simulink model "MATLAB Simulink Model"  (R2020b)
settings: Solver=ode4  StartTime=0.0  StopTime=1  RelTol=1e-3
InitFcn:
  | clear;
  | clc;
  | 
  | %Motor Parameters
  | r1 = 1.405;
  | l1  = 0.005839;
  | r2 = 1.395;
  | l2 = 0.005839;
  | Lm = 0.1722;
  | 
  | %Motor Rated Values
  | Vrat = 400;
  | frat = 50;
  | 
  | x1 = 2*pi*frat*l1;
  | x2 = 2*pi*frat*l2;
  | Xm = 2*pi*frat*Lm;
  | Prat = 4*1000;
  | Nrat = 1430;
  | Ns = 120*frat/4;
  | nrat = Nrat*2*pi/60;
  | ns = Ns*2*pi/60;
  | srat = (Ns-Nrat)/Ns;
  | 
  | E1 = Vrat/sqrt(3); %phase voltage
  | IL = E1/( (r1 + (1i*x1) ) + ( ( (1i*x2) +(r2/srat) )*1i*Xm / ( (1i*Xm) + (1i*x2) + (r2/srat) ) ) );
  | E2 = E1 - (IL*(r1 + (1i*x1) ) );
  | Trat = (3/(ns))*srat*abs(E2)*abs(E2)*r2/((r2*r2) + (srat*srat*x2*x2));
  | %Trat = Prat/nrat;
  | 
  | %System Variables
  | Tsys = (1e-6);
  | Ts = (100e-6);
  | freq = 50;
  | 
  | m=1*freq/50;
  | %m = 1 * (freq/50);
  | Vbus = (400*sqrt(2)*2/sqrt(3)) / (1.15);
  | 
  | Vref = (Vbus*sqrt(3)/2) * m;
  | delay = Ts/Tsys;
  | 
  | % Motor Starting Parameters
  | inc_time = 0.1;
  | 
  | %Motor Loading time
  | load_time = 0.5;
  | 
  | %No. of Hybrid Zones
  | numzones = 3;
  | 
  | %Load ML model Weights
  | 
  | W1R_s1 = readmatrix('Regression Weights\W1_subnet1_tmp_odd_90.xlsx');
  | b1R_s1 = readmatrix('Regression Weights\b1_subnet1_tmp_odd_90.xlsx');
  | W1R_s2 = readmatrix('Regression Weights\W1_subnet2_tmp_odd_90.xlsx');
  | b1R_s2 = readmatrix('Regression Weights\b1_subnet2_tmp_odd_90.xlsx');
  | 
  | W2R = readmatrix('Regression Weights\W2_subnet_tmp_odd_90.xlsx');
  | b2R = readmatrix('Regression Weights\b2_subnet_tmp_odd_90.xlsx');
  | ... (+9 lines)
libraries: powerlib x72, simulink x55, powerlib_meascontrol x15, dspstat3 x11, dspsigops x1
(part 4 of 5)

== system MATLAB Simulink Model/Space Vector PWM based VSI 1/Gating Pulse Generator/Gate Pulse Generator for 2721 Sequence/For Even Sector ==
  "S1, S3, S5" : Inport
  AND : Logic  IconShape=distinctive  AllPortsSameDT=off  OutDataTypeStr=boolean
  AND1 : Logic  IconShape=distinctive  AllPortsSameDT=off  OutDataTypeStr=boolean
  AND2 : Logic  IconShape=distinctive  AllPortsSameDT=off  OutDataTypeStr=boolean
  Carrier1 : simulink/Sources/Repeating Sequence  rep_seq_t=[0 Ts/2 Ts]  rep_seq_y=[Ts-(1e-16) 0 Ts-(1e-16)]
  Carrier2 : simulink/Sources/Repeating Sequence  rep_seq_t=[0 Ts/2 Ts]  rep_seq_y=[0 Ts-(1e-16) 0]
  Constant : Constant
  Constant1 : Constant  Value=2
  Constant2 : Constant  Value=3
  Demux : Demux  Outputs=3
  GreaterThan{,1..3} (4 alike) : RelationalOperator  OutDataTypeStr=boolean  RndMeth=Simplest
  GreaterThan4 : RelationalOperator  Operator===  OutDataTypeStr=boolean  RndMeth=Simplest
  GreaterThan5 : RelationalOperator  Operator===  OutDataTypeStr=boolean  RndMeth=Simplest
  GreaterThan6 : RelationalOperator  Operator===  OutDataTypeStr=boolean  RndMeth=Simplest
  MATLAB Function : MATLAB Function  TreatAsAtomicUnit=on
  XOR : Logic  Operator=XOR  IconShape=distinctive  AllPortsSameDT=off  OutDataTypeStr=boolean
  XOR1 : Logic  Operator=XOR  IconShape=distinctive  AllPortsSameDT=off  OutDataTypeStr=boolean
  XOR2 : Logic  Operator=XOR  IconShape=distinctive  AllPortsSameDT=off  OutDataTypeStr=boolean
  Gate 1 Pulse : Outport
  Gate 3 Pulse : Outport  Port=2
  Gate 5 Pulse : Outport  Port=3
  wires:
  Constant1/1 -> GreaterThan5/1
  AND2/1 -> XOR2/2
  MATLAB Function/3(S5) -> GreaterThan2/1
  XOR1/1 -> Gate 3 Pulse/1
  GreaterThan/1 -> XOR/1
  GreaterThan5/1 -> AND1/2
  MATLAB Function/5(addidx) -> GreaterThan4/2, GreaterThan5/2, GreaterThan6/2
  Constant/1 -> GreaterThan4/1
  Carrier1/1 -> GreaterThan2/2, GreaterThan1/2, GreaterThan/2
  XOR/1 -> Gate 1 Pulse/1
  MATLAB Function/4(addtime) -> GreaterThan3/1
  MATLAB Function/2(S3) -> GreaterThan1/1
  AND1/1 -> XOR1/2
  Constant2/1 -> GreaterThan6/1
  GreaterThan4/1 -> AND/2
  GreaterThan3/1 -> AND2/1, AND1/1, AND/1
  GreaterThan1/1 -> XOR1/1
  GreaterThan6/1 -> AND2/2
  XOR2/1 -> Gate 5 Pulse/1
  Carrier2/1 -> GreaterThan3/2
  Demux/3 -> MATLAB Function/3("S5 ")
  Demux/2 -> MATLAB Function/2("S3 ")
  Demux/1 -> MATLAB Function/1("S1 ")
  MATLAB Function/1(S1) -> GreaterThan/1
  "S1, S3, S5"/1 -> Demux/1
  GreaterThan2/1 -> XOR2/1
  AND/1 -> XOR/2

== system MATLAB Simulink Model/Space Vector PWM based VSI 1/Gating Pulse Generator/Gate Pulse Generator for 2721 Sequence/For Odd Sector ==
  "S1, S3, S1" : Inport
  AND3 : Logic  IconShape=distinctive  AllPortsSameDT=off  OutDataTypeStr=boolean
  AND4 : Logic  IconShape=distinctive  AllPortsSameDT=off  OutDataTypeStr=boolean
  AND5 : Logic  IconShape=distinctive  AllPortsSameDT=off  OutDataTypeStr=boolean
  Carrier3 : simulink/Sources/Repeating Sequence  rep_seq_t=[0 Ts/2 Ts]  rep_seq_y=[0 Ts-(1e-16) 0]
  Constant3 : Constant
  Constant4 : Constant  Value=2
  Constant5 : Constant  Value=3
  Demux1 : Demux  Outputs=3
  GreaterThan{7..10} (4 alike) : RelationalOperator  OutDataTypeStr=boolean  RndMeth=Simplest
  GreaterThan11 : RelationalOperator  Operator===  OutDataTypeStr=boolean  RndMeth=Simplest
  GreaterThan12 : RelationalOperator  Operator===  OutDataTypeStr=boolean  RndMeth=Simplest
  GreaterThan13 : RelationalOperator  Operator===  OutDataTypeStr=boolean  RndMeth=Simplest
  MATLAB Function1 : MATLAB Function  TreatAsAtomicUnit=on
  XOR3 : Logic  Operator=XOR  IconShape=distinctive  AllPortsSameDT=off  OutDataTypeStr=boolean
  XOR4 : Logic  Operator=XOR  IconShape=distinctive  AllPortsSameDT=off  OutDataTypeStr=boolean
  XOR5 : Logic  Operator=XOR  IconShape=distinctive  AllPortsSameDT=off  OutDataTypeStr=boolean
  Gate 1 Pulse : Outport
  Gate 3 Pulse : Outport  Port=2
  Gate 5 Pulse : Outport  Port=3
  wires:
  MATLAB Function1/4(subtime) -> GreaterThan10/1
  Carrier3/1 -> GreaterThan9/2, GreaterThan10/2, GreaterThan8/2, GreaterThan7/2
  "S1, S3, S1"/1 -> Demux1/1
  XOR3/1 -> Gate 1 Pulse/1
  Constant3/1 -> GreaterThan11/1
  XOR5/1 -> Gate 5 Pulse/1
  Demux1/3 -> MATLAB Function1/3("S5 ")
  XOR4/1 -> Gate 3 Pulse/1
  GreaterThan7/1 -> XOR3/1
  Constant5/1 -> GreaterThan13/1
  GreaterThan13/1 -> AND5/2
  GreaterThan8/1 -> XOR4/1
  MATLAB Function1/1(S1) -> GreaterThan7/1
  AND3/1 -> XOR3/2
  GreaterThan11/1 -> AND3/2
  Demux1/1 -> MATLAB Function1/1("S1 ")
  AND4/1 -> XOR4/2
  Demux1/2 -> MATLAB Function1/2("S3 ")
  AND5/1 -> XOR5/2
  MATLAB Function1/2(S3) -> GreaterThan8/1
  MATLAB Function1/5(subidx) -> GreaterThan11/2, GreaterThan12/2, GreaterThan13/2
  GreaterThan10/1 -> AND5/1, AND4/1, AND3/1
  MATLAB Function1/3(S5) -> GreaterThan9/1
  Constant4/1 -> GreaterThan12/1
  GreaterThan9/1 -> XOR5/1
  GreaterThan12/1 -> AND4/2

== system MATLAB Simulink Model/Space Vector PWM based VSI 1/Gating Pulse Generator/Gate Pulse Generator for 7212 Sequence/For Even Sector ==
  "S1, S3, S1" : Inport
  AND3 : Logic  IconShape=distinctive  AllPortsSameDT=off  OutDataTypeStr=boolean
  AND4 : Logic  IconShape=distinctive  AllPortsSameDT=off  OutDataTypeStr=boolean
  AND5 : Logic  IconShape=distinctive  AllPortsSameDT=off  OutDataTypeStr=boolean
  Carrier3 : simulink/Sources/Repeating Sequence  rep_seq_t=[0 Ts/2 Ts]  rep_seq_y=[Ts-(1e-16) 0 Ts-(1e-16)]
  Constant3 : Constant
  Constant4 : Constant  Value=2
  Constant5 : Constant  Value=3
  Demux1 : Demux  Outputs=3
  GreaterThan{7..10} (4 alike) : RelationalOperator  OutDataTypeStr=boolean  RndMeth=Simplest
  GreaterThan11 : RelationalOperator  Operator===  OutDataTypeStr=boolean  RndMeth=Simplest
  GreaterThan12 : RelationalOperator  Operator===  OutDataTypeStr=boolean  RndMeth=Simplest
  GreaterThan13 : RelationalOperator  Operator===  OutDataTypeStr=boolean  RndMeth=Simplest
  MATLAB Function1 : MATLAB Function  TreatAsAtomicUnit=on
  XOR3 : Logic  Operator=XOR  IconShape=distinctive  AllPortsSameDT=off  OutDataTypeStr=boolean
  XOR4 : Logic  Operator=XOR  IconShape=distinctive  AllPortsSameDT=off  OutDataTypeStr=boolean
  XOR5 : Logic  Operator=XOR  IconShape=distinctive  AllPortsSameDT=off  OutDataTypeStr=boolean
  Gate 1 Pulse : Outport
  Gate 3 Pulse : Outport  Port=2
  Gate 5 Pulse : Outport  Port=3
  wires:
  GreaterThan12/1 -> AND4/2
  Carrier3/1 -> GreaterThan9/2, GreaterThan10/2, GreaterThan8/2, GreaterThan7/2
  "S1, S3, S1"/1 -> Demux1/1
  GreaterThan9/1 -> XOR5/1
  Constant4/1 -> GreaterThan12/1
  GreaterThan10/1 -> AND5/1, AND4/1, AND3/1
  MATLAB Function1/1(S1) -> GreaterThan7/1
  MATLAB Function1/3(S5) -> GreaterThan9/1
  MATLAB Function1/5(subidx) -> GreaterThan11/2, GreaterThan12/2, GreaterThan13/2
  Demux1/1 -> MATLAB Function1/1("S1 ")
  MATLAB Function1/2(S3) -> GreaterThan8/1
  Constant3/1 -> GreaterThan11/1
  Constant5/1 -> GreaterThan13/1
  GreaterThan13/1 -> AND5/2
  AND5/1 -> XOR5/2
  MATLAB Function1/4(subtime) -> GreaterThan10/1
  AND3/1 -> XOR3/2
  AND4/1 -> XOR4/2
  XOR4/1 -> Gate 3 Pulse/1
  GreaterThan8/1 -> XOR4/1
  Demux1/2 -> MATLAB Function1/2("S3 ")
  GreaterThan11/1 -> AND3/2
  GreaterThan7/1 -> XOR3/1
  Demux1/3 -> MATLAB Function1/3("S5 ")
  XOR5/1 -> Gate 5 Pulse/1
  XOR3/1 -> Gate 1 Pulse/1

== system MATLAB Simulink Model/Space Vector PWM based VSI 1/Gating Pulse Generator/Gate Pulse Generator for 7212 Sequence/For Odd Sector ==
  "S1, S3, S5" : Inport
  AND : Logic  IconShape=distinctive  AllPortsSameDT=off  OutDataTypeStr=boolean
  AND1 : Logic  IconShape=distinctive  AllPortsSameDT=off  OutDataTypeStr=boolean
  AND2 : Logic  IconShape=distinctive  AllPortsSameDT=off  OutDataTypeStr=boolean
  Carrier1 : simulink/Sources/Repeating Sequence  rep_seq_t=[0 Ts/2 Ts]  rep_seq_y=[0 Ts-(1e-16) 0]
  Carrier2 : simulink/Sources/Repeating Sequence  rep_seq_t=[0 Ts/2 Ts]  rep_seq_y=[Ts-(1e-16) 0 Ts-(1e-16)]
  Constant : Constant
  Constant1 : Constant  Value=2
  Constant2 : Constant  Value=3
  Demux : Demux  Outputs=3
  GreaterThan{,1..3} (4 alike) : RelationalOperator  OutDataTypeStr=boolean  RndMeth=Simplest
  GreaterThan4 : RelationalOperator  Operator===  OutDataTypeStr=boolean  RndMeth=Simplest
  GreaterThan5 : RelationalOperator  Operator===  OutDataTypeStr=boolean  RndMeth=Simplest
  GreaterThan6 : RelationalOperator  Operator===  OutDataTypeStr=boolean  RndMeth=Simplest
  MATLAB Function : MATLAB Function  TreatAsAtomicUnit=on
  XOR : Logic  Operator=XOR  IconShape=distinctive  AllPortsSameDT=off  OutDataTypeStr=boolean
  XOR1 : Logic  Operator=XOR  IconShape=distinctive  AllPortsSameDT=off  OutDataTypeStr=boolean
  XOR2 : Logic  Operator=XOR  IconShape=distinctive  AllPortsSameDT=off  OutDataTypeStr=boolean
  Gate 1 Pulse : Outport
  Gate 3 Pulse : Outport  Port=2
  Gate 5 Pulse : Outport  Port=3
  wires:
  GreaterThan6/1 -> AND2/2
  Demux/2 -> MATLAB Function/2("S3 ")
  Demux/1 -> MATLAB Function/1("S1 ")
  Demux/3 -> MATLAB Function/3("S5 ")
  MATLAB Function/5(addidx) -> GreaterThan4/2, GreaterThan5/2, GreaterThan6/2
  XOR1/1 -> Gate 3 Pulse/1
  Constant1/1 -> GreaterThan5/1
  AND2/1 -> XOR2/2
  AND/1 -> XOR/2
  "S1, S3, S5"/1 -> Demux/1
  Constant2/1 -> GreaterThan6/1
  GreaterThan5/1 -> AND1/2
  GreaterThan2/1 -> XOR2/1
  Carrier2/1 -> GreaterThan3/2
  MATLAB Function/1(S1) -> GreaterThan/1
  GreaterThan4/1 -> AND/2
  XOR2/1 -> Gate 5 Pulse/1
  GreaterThan1/1 -> XOR1/1
  GreaterThan3/1 -> AND2/1, AND1/1, AND/1
  AND1/1 -> XOR1/2
  GreaterThan/1 -> XOR/1
  MATLAB Function/4(addtime) -> GreaterThan3/1
  Constant/1 -> GreaterThan4/1
  MATLAB Function/3(S5) -> GreaterThan2/1
  XOR/1 -> Gate 1 Pulse/1
  MATLAB Function/2(S3) -> GreaterThan1/1
  Carrier1/1 -> GreaterThan2/2, GreaterThan1/2, GreaterThan/2

== matlab function MATLAB Simulink Model/3 Phase Induction Machine/Angle Calculation/MATLAB Function ==
  data: wold input; wnew output; wTs input
function wnew = fcn(wold, wTs)
    wnew = rem(wold + wTs, 2*pi);
end

== matlab function MATLAB Simulink Model/Space Vector PWM based VSI /Gate Pulse Generator/Gate Pulse Values ==
  data: count output; count input; G1 output size=1; S1 input; S3 input; S5 input; G3 output size=1; G5 output size=1; Ts input; Tsys input
function [count, G1, G3, G5] = fcn(count, S1, S3, S5, Ts, Tsys)
    count = double(rem(int32(1+count), int32(Ts/Tsys)));
    G1 = S1(1+count);
    G3 = S3(1+count);
    G5 = S5(1+count);
    
%     G1=S1;
%     G3= S3;
%     G5 = S5;
end

== matlab function MATLAB Simulink Model/Space Vector PWM based VSI /Gating Pulse Generator/Gate Pulse Generator for 0127 Sequence 1/For Odd Sector/MATLAB Function1 ==
  data: S1 input; S1 output; S3 input; S5 input; S3 output; S5 output; subtime output; subidx output
function [S1, S3, S5, subtime,subidx] = fcn(S1, S3, S5)
    S = [S1 S3 S5];
    [~, idx] = mink([S1 S3 S5], 3);
    
    subtime = ( ( S(idx(2)) - S(idx(1)) )/2);
    S(idx(1)) = S(idx(1)) + subtime;
    subidx = idx(1);
    
    S1 = S(1);
    S3 = S(2);
    S5 = S(3);
end

== matlab function MATLAB Simulink Model/Space Vector PWM based VSI /Gating Pulse Generator/Gate Pulse Generator for 7212 Sequence/For Even Sector/MATLAB Function1 ==
  data: S1 input; S1 output; S3 input; S5 input; S3 output; S5 output; subtime output; subidx output
function [S1, S3, S5, subtime,subidx] = fcn(S1, S3, S5)
    S = [S1 S3 S5];
    [~, idx] = mink([S1 S3 S5], 3);
    
    S(idx(2)) = (S(idx(2)) + S(idx(3)))/2;
    
    subidx = idx(2);
    subtime = S(idx(3)) - S(idx(2));
    
    S1 = S(1);
    S3 = S(2);
    S5 = S(3);
end

== matlab function MATLAB Simulink Model/Space Vector PWM based VSI /Gating Pulse Generator/Gate Pulse Generator for 0121 Sequence/For Even Sector/MATLAB Function ==
  data: S1 input; S1 output; S3 input; S5 input; S3 output; S5 output; addtime output; addidx output
function [S1, S3, S5, addtime,addidx] = fcn(S1, S3, S5)
    S = [S1 S3 S5];
    [~, idx] = mink([S1 S3 S5], 3);
    
    addtime = (S(idx(2)) - S(idx(1)))/2;
    addidx = idx(2);
    S(idx(2)) = S(idx(2)) - addtime;
    
    S1 = S(1);
    S3 = S(2);
    S5 = S(3);
end

== matlab function MATLAB Simulink Model/Space Vector PWM based VSI /Switching Times and Sector/Switch Times and Sequence Calculation ==
  data: Vref input; angle input; Ts input; Vbus input; sector output
function sector  = fcn(Vref, angle, Ts, Vbus)
    
    numzones = 3;
    %     Using ML Models 
    m = (2/sqrt(3))*(Vref/Vbus);
    theta = rem(angle, (pi/3));
    flag = 0;
    if numzones == 1
        flag = 1;
    end
    
    %Switching times calculation of different vectors
    if m <= 1                % Linear modulation (Overmodulation mode 0)
        n2 = Vref*cos( theta );
        n1 = Vref*cos( (pi/3) - theta );

        T1 = (2*Ts/(3*Vbus)) * ((-n1) + (2*n2));
        T2 = (2*Ts/(3*Vbus)) * ((2*n1) - n2);
        T0 = Ts-(T1+T2);
        flag = 1;
        
    elseif m<=1.05      % Overmodulation mode I
        alpha_t = (pi/6) - acos(1/m);
        alpha_t = alpha_t/2;
        if theta > alpha_t && theta < (pi/3) - alpha_t
            T1 = (sin( (pi/3) - theta ) / ( sin( (pi/3) - theta ) + sin( theta ) ) ) * Ts;
            T2 = Ts-T1;
            T0=0;
        else
            n2 = Vref*cos( theta );
            n1 = Vref*cos( (pi/3) - theta );
            T1 = (2*Ts/(3*Vbus)) * ((-n1) + (2*n2));
            T2 = (2*Ts/(3*Vbus)) * ((2*n1) - n2);
            T0 = Ts-(T1+T2);
            flag = 1;
        end
        
    elseif m <= 1.10    % Overmodulation mode II
        alpha_h = (pi/6) - acos(1/m);
        if theta <= alpha_h
            T1 = Ts;
            T2=0;
            T0=0;
            
        elseif theta > alpha_h && theta < (pi/3) - alpha_h
            T1 = (sin( (pi/3) - theta ) / ( sin( (pi/3) - theta ) + sin( theta ) ) ) * Ts;
            T2 = Ts-T1;
            T0=0;
            
        else
            T1 = 0;
            T2 = Ts;
            T0 = 0;
        end
        
    else        % Six Step Mode
        if theta <= (pi/6)
            T1 = Ts;
            T2 = 0;
            T0 = 0;
        else
            T1 = 0;
            T2 = Ts;
            T0 = 0;
        end
        
    end
    
    if flag == 1
        % Switching Sequence Determination
        Q1 = (cos(theta) - (Vref/Vbus)) * T1;
        Q2 = (cos( (pi/3) - theta) - (Vref/Vbus)) * T2;
        Q0 = - (Vref/Vbus)*T0;
        D = sin(theta) * T1;

        %Error Functions (Squared) for Different Switching Sequences
        F_0127 = ( (1/3) * ( (0.5*Q0).^2 ) * T0 / (2*Ts) ) + ( (1/3) * ( ( (0.5*Q0).^2 ) + ( 0.5*Q0* ( (0.5*Q0) + Q1 ) ) + ( ( 1* ( (0.5*Q0) + Q1 ) ).^2) ) * (T1/Ts) ) + ( (1/3) * ( ( ( (0.5*Q0) + Q1).^2) - ( ( (0.5*Q0) + Q1) * (0.5*Q0) ) + ( (0.5*Q0).^2 ) ) * (T2/Ts) ) + ( (1/3) * ( (0.5*Q0).^2 ) * ( T0 / (2*Ts) ) ) + ( (1/3) * (D.^2) * ( (T1+T2) / Ts ) );

        F_012 = ( (4/27) * (Q0.^2) * (T0/Ts) ) + ( (4/27) * ( (Q0.^2) + ( Q0*(Q0+Q1) ) + ( (Q0+Q1).^2 ) ) * (T1/Ts) ) + ( (4/27) * ( (Q0+Q1).^2 ) * (T2/Ts) ) + ( (4/27) * (D.^2) * ( (T1+T2) / Ts) );

        F_721 = ( (4/27) * (Q0.^2) * (T0/Ts) ) + ( (4/27) * ( (Q0.^2) + ( Q0*(Q0+Q2) ) + ( (Q0+Q2).^2 ) ) * (T2/Ts) ) + ( (4/27) * ( (Q0+Q2).^2 ) * (T1/Ts) ) + ( (4/27) * (D.^2) * ( (T1+T2) / Ts) );

        F_0121 = ( (1/3) * (Q0.^2) * (T0/Ts) ) + ( (1/3) * ( (Q0.^2) + ( Q0*( Q0 + (0.5*Q1) ) ) + ( ( Q0 + (0.5*Q1) ).^2 ) ) * ( T1 / (2*Ts) ) ) + ( (1/3) * ( ( ( Q0 + (0.5*Q1) ).^2 ) - ( ( Q0 + (0.5*Q1) ) * (0.5*Q1) ) + ( (0.5*Q1).^2 ) ) * (T2/Ts) ) + ( (1/3) * ( (0.5*Q1).^2 ) * (T1 / (2*Ts) ) ) + ( (1/3) * ( (0.5*D).^2 ) * ( (T1+T2) / Ts ) );

        F_7212 = ( (1/3) * (Q0.^2) * (T0/Ts) ) + ( (1/3) * ( (Q0.^2) + ( Q0*( Q0 + (0.5*Q2) ) ) + ( ( Q0 + (0.5*Q2) ).^2 ) ) * ( T2 / (2*Ts) ) ) + ( (1/3) * ( ( ( Q0 + (0.5*Q2) ).^2 ) - ( ( Q0 + (0.5*Q2) ) * (0.5*Q2) ) + ( (0.5*Q2).^2 ) ) * (T1/Ts) ) + ( (1/3) * ( (0.5*Q2).^2 ) * (T2 / (2*Ts) ) ) + ( (1/3) * ( (0.5*D).^2 ) * ( (T1+T2) / Ts ) );

        F_1012 = ( (1/3) * ( ( 0.5*Q1).^2 ) * (T1 / (2*Ts) ) ) + ( (1/3) * ( ( (0.5*Q1).^2 ) + ( 0.5*Q1*( (0.5*Q1) + Q0 ) ) + ( ( (0.5*Q1) + Q0 ).^2 ) ) * (T0/Ts) ) + ( (1/3) * ( ( ( (0.5*Q1) + Q0 ).^2 ) - ( ( (0.5*Q1) + Q0 )*Q2 ) + (Q2.^2) ) * ( T1 / (2*Ts) ) ) + ( (1/3) * (Q2.^2) * (T2/Ts) ) + ( (1/3) * ( (0.5*D).^2 ) * ( T1 / (2*Ts) ) ) + ( ( (0.5*D).^2 ) * (T0/Ts) ) + ( (1/3) * ( ( (0.5*D).^2 ) + ( (0.5*D) * D ) + (D.^2) ) * ( T1 / (2*Ts) ) ) + ( (1/3) * (D.^2) * (T2/Ts) );

        F_2721 = ( (1/3) * ( ( 0.5*Q2).^2 ) * (T2 / (2*Ts) ) ) + ( (1/3) * ( ( (0.5*Q2).^2 ) + ( 0.5*Q2*( (0.5*Q2) + Q0 ) ) + ( ( (0.5*Q2) + Q0 ).^2 ) ) * (T0/Ts) ) + ( (1/3) * ( ( ( (0.5*Q2) + Q0 ).^2 ) - ( ( (0.5*Q2) + Q0 )*Q1 ) + (Q1.^2) ) * ( T2 / (2*Ts) ) ) + ( (1/3) * (Q1.^2) * (T1/Ts) ) + ( (1/3) * ( (0.5*D).^2 ) * ( T2 / (2*Ts) ) ) + ( ( (0.5*D).^2 ) * (T0/Ts) ) + ( (1/3) * ( ( (0.5*D).^2 ) + ( (0.5*D) * D ) + (D.^2) ) * ( T2 / (2*Ts) ) ) + ( (1/3) * (D.^2) * (T1/Ts) );
        
        if numzones == 1
            F = [F_0127];
            
        elseif numzones == 3
            %For Three Zone Hybrid PWM
            F = [F_0127, F_0121, F_7212];
            
        elseif numzones == 5
            %For Five Zone Hybrid PWM
            F = [F_0127, F_0121, F_7212, F_1012, F_2721];
        
        elseif numzones == 7
            %For Seven Zone Hybrid PWM
            F = [F_0127, F_0121, F_7212, F_1012, F_2721, F_012, F_721];
            
        else
            F = F_0127;
        end
        
        [~, idx] = min(F);

        if idx == 1
            switchseq = "0127";
        elseif idx == 2
            switchseq = "0121";
        elseif idx == 3
            switchseq = "7212";
        elseif idx == 4
            switchseq = "1012";
        elseif idx == 5
            switchseq = "2721";
        elseif idx == 6
            switchseq = "012";
        elseif idx == 7
            switchseq = "721";
        else
            switchseq = "0127";
        end
        
    else
        if theta < (pi/6)
            switchseq = "0121";
        else
            switchseq = "7212";
        end
    end
    
    % Switching Times calculation of switches
    Vsamp = Vref*exp(1i*angle);
    
    V1 = Vbus*exp(1i*0);
    V2 = Vbus*exp(1i*(pi/3));
    V3 = Vbus*exp(1i*(2*pi/3));
    V4 = Vbus*exp(1i*(3*pi/3));
    V5 = Vbus*exp(1i*(4*pi/3));
    V6 = Vbus*exp(1i*(5*pi/3));

    V = [V1; V2; V3; V4; V5; V6];
    V = V - Vsamp;
    [~, minVidx] = mink(V, 2);

%         minVidx = minVidx(:, 1);

    if max(minVidx) == 6 && min(minVidx) == 1
        minVidx = 6;
    else
        minVidx = min(minVidx);
    end
    
    sector = minVidx;
    
    if switchseq == "0127"
        swseq = 1;
    elseif switchseq == "0121"
        swseq = 2;
    elseif switchseq == "7212"
        swseq = 3;
    elseif switchseq == "1012"
        swseq = 4;
    elseif switchseq == "2721"
        swseq = 5;
    elseif switchseq == "012"
        swseq = 6;
    elseif switchseq == "721"
        swseq = 7;
    else
        swseq = 1;
    end
%     
%     %Using NN to predict switch times
%     
%     %Loading Necessary weight matrices
%     W1 = evalin('base', 'W1R');
%     b1 = evalin('base', 'b1R');
%     W2 = evalin('base', 'W2R');
%     b2 = evalin('base', 'W2R');
%     
%     %Predicting Switch Times
%     X = [m angle];
% %     y1 = zeros(1, size(b1, 1));
% %     y2 = zeros(1, size(b2, 2));
%     
%     y = X*(W1');
%     y = y + b1';      %Passing through 1st Layer (Hidden)
%     y = tanh(y);                  %Applying Activation Function (tanh)
%     
%     y = y*W2';
%     y = y+b2';        %Passing through 2nd Layer (Output)
%     y = 1./(1+exp(-y));      %Applying Activation Function (sigmoid)
%     
%     %Allocating Switch Times
%     S1 = y(1)*Ts;
%     S3 = y(2)*Ts;
%     S5 = y(3)*Ts;
    
end

== matlab function MATLAB Simulink Model/Space Vector PWM based VSI /Gating Pulse Generator/Gate Pulse Generator for 1012 Sequence/For Even Sector/MATLAB Function1 ==
  data: S1 input; S1 output; S3 input; S5 input; S3 output; S5 output; subtime output; subidx output
function [S1, S3, S5, subtime,subidx] = fcn(S1, S3, S5)
    S = [S1 S3 S5];
    [~, idx] = mink([S1 S3 S5], 3);
    
    subtime = ( ( S(idx(2)) - S(idx(1)) )/2);
    S(idx(1)) = S(idx(1)) + subtime;
    subidx = idx(1);
    
    S1 = S(1);
    S3 = S(2);
    S5 = S(3);
end

== matlab function MATLAB Simulink Model/Space Vector PWM based VSI /Gating Pulse Generator/Gate Pulse Generator for 0127 Sequence 1/For Even Sector/MATLAB Function ==
  data: S1 input; S1 output; S3 input; S5 input; S3 output; S5 output; addtime output; addidx output
function [S1, S3, S5, addtime,addidx] = fcn(S1, S3, S5)
    S = [S1 S3 S5];
    [~, idx] = mink([S1 S3 S5], 3);
    
    addtime = (S(idx(3)) - S(idx(2)))/2;
    addidx = idx(3);
    S(idx(3)) = S(idx(3)) - addtime;
    
    S1 = S(1);
    S3 = S(2);
    S5 = S(3);
end

== matlab function MATLAB Simulink Model/Space Vector PWM based VSI /Gating Pulse Generator/Gate Pulse Generator for 0121 Sequence/For Odd Sector/MATLAB Function ==
  data: S1 input; S1 output; S3 input; S5 input; S3 output; S5 output; subtime output; subidx output
function [S1, S3, S5, subtime,subidx] = fcn(S1, S3, S5)
    S = [S1 S3 S5];
    [~, idx] = mink([S1 S3 S5], 3);
    
    S(idx(2)) = (S(idx(2)) + S(idx(3)))/2;
    
    subidx = idx(2);
    subtime = S(idx(3)) - S(idx(2));
    
    S1 = S(1);
    S3 = S(2);
    S5 = S(3);
end

== matlab function MATLAB Simulink Model/Space Vector PWM based VSI /Gating Pulse Generator/Gate Pulse Generator for 1012 Sequence/For Odd Sector/MATLAB Function ==
  data: S1 input; S1 output; S3 input; S5 input; S3 output; S5 output; addtime output; addidx output
function [S1, S3, S5, addtime,addidx] = fcn(S1, S3, S5)
    S = [S1 S3 S5];
    [~, idx] = mink([S1 S3 S5], 3);
    
    addtime = (S(idx(3)) - S(idx(2)))/2;
    addidx = idx(3);
    S(idx(3)) = S(idx(3)) - addtime;
    
    S1 = S(1);
    S3 = S(2);
    S5 = S(3);
end

== matlab function MATLAB Simulink Model/Space Vector PWM based VSI /Gating Pulse Generator/Gate Pulse Generator for 2721 Sequence/For Even Sector/MATLAB Function ==
  data: S1 input; S1 output; S3 input; S5 input; S3 output; S5 output; addtime output; addidx output
function [S1, S3, S5, addtime,addidx] = fcn(S1, S3, S5)
    S = [S1 S3 S5];
    [~, idx] = mink([S1 S3 S5], 3);
    
    addtime = (S(idx(3)) - S(idx(2)))/2;
    addidx = idx(3);
    S(idx(3)) = S(idx(3)) - addtime;
    
    S1 = S(1);
    S3 = S(2);
    S5 = S(3);
end

== matlab function MATLAB Simulink Model/15 Hz System/Space Vector PWM based VSI 1/Switching Times and Sector/Switching times of all switches ==
  data: Vref input; S1 output; theta input; Ts input; sector input; S3 output; S5 output; Vbus input
function [S1, S3, S5] = fcn(Vref, theta, Ts, sector, Vbus)
    n2 = Vref*cos(theta);
    n1 = Vref*cos((pi/3)-theta);
    
%     T1 = sqrt(3)*Ts*Vref*(sin(sector*pi/3)*cos(angle - ((sector-1)*pi/3)) - cos(sector*pi/3)*sin(angle - ((sector-1)*pi/3)))/u(3);
%     T2 = sqrt(3)*Ts*Vref*(-cos(angle - ((sector-1)*pi/3))*sin((sector-1)*pi/3) + sin(angle - ((sector-1)*pi/3))*cos((sector-1)*pi/3))/u(3);
    
    T1 = (2*Ts/(3*Vbus)) * ((-n1) + (2*n2));
    T2 = (2*Ts/(3*Vbus)) * ((2*n1) - n2);
    T0 = Ts-(T1+T2);
  
    if sector == 1
        S1 = T1+T2+(T0/2);
%         S4 = T0/2;
        S3 = T2+(T0/2);
%         S6 = T1+(T0/2);
        S5 = T0/2;
%         S2 = T1+T2+(T0/2);
    elseif sector == 2
        S1 = T1+(T0/2);
%         S4 = T2+(T0/2);
        S3 = T1+T2+(T0/2);
%         S6 = (T0/2);
        S5 = T0/2;
%         S2 = T1+T2+(T0/2);
    elseif sector == 3
        S1 = (T0/2);
%         S4 = T1+T2+(T0/2);
        S3 = T1+T2+(T0/2);
%         S6 = (T0/2);
        S5 = T2+(T0/2);
%         S2 = T1+(T0/2);
    elseif sector == 4
        S1 = (T0/2);
%         S4 = T1+T2+(T0/2);
        S3 = T1+(T0/2);
%         S6 = T2+(T0/2);
        S5 = T1+T2+(T0/2);
%         S2 = (T0/2);
    elseif sector == 5
        S1 = T2+(T0/2);
%         S4 = T1+(T0/2);
        S3 = (T0/2);
%         S6 = T1+T2+(T0/2);
        S5 = T1+T2+(T0/2);
%         S2 = (T0/2);
    elseif sector == 6
        S1 = T1+T2+(T0/2);
%         S4 = T0/2;
        S3 = (T0/2);
%         S6 = T1+T2+(T0/2);
        S5 = T1+(T0/2);
%         S2 = T2+(T0/2);
    else
        S1 = (T1+T2+T0)/2;
        S3 = (T1+T2+T0)/2;
        S5 = (T1+T2+T0)/2;
    end
end

== matlab function MATLAB Simulink Model/Space Vector PWM based VSI /Switching Times and Sector/MATLAB Function1 ==
  data: u input; S1 output; S3 output; S5 output
function [S1, S3, S5] = fcn(u)
    S1 = u(1);
    S3 = u(2);
    S5 = u(3);
end

== matlab function MATLAB Simulink Model/Space Vector PWM based VSI /Gating Pulse Generator/Gate Pulse Generator for 7212 Sequence/For Odd Sector/MATLAB Function ==
  data: S1 input; S1 output; S3 input; S5 input; S3 output; S5 output; addtime output; addidx output
function [S1, S3, S5, addtime,addidx] = fcn(S1, S3, S5)
    S = [S1 S3 S5];
    [~, idx] = mink([S1 S3 S5], 3);
    
    addtime = (S(idx(2)) - S(idx(1)))/2;
    addidx = idx(2);
    S(idx(2)) = S(idx(2)) - addtime;
    
    S1 = S(1);
    S3 = S(2);
    S5 = S(3);
end

== matlab function MATLAB Simulink Model/Space Vector PWM based VSI /Gating Pulse Generator/Gate Pulse Generator for 2721 Sequence/For Odd Sector/MATLAB Function1 ==
  data: S1 input; S1 output; S3 input; S5 input; S3 output; S5 output; subtime output; subidx output
function [S1, S3, S5, subtime,subidx] = fcn(S1, S3, S5)
    S = [S1 S3 S5];
    [~, idx] = mink([S1 S3 S5], 3);
    
    subtime = ( ( S(idx(2)) - S(idx(1)) )/2);
    S(idx(1)) = S(idx(1)) + subtime;
    subidx = idx(1);
    
    S1 = S(1);
    S3 = S(2);
    S5 = S(3);
end

== matlab function MATLAB Simulink Model/Space Vector PWM based VSI /Switching Times and Sector/Feature Expand ==
  data: X input; new_X output size=[1 18]
function new_X = fcn(X)
    X = X';
    new_X = zeros(1,18);
    new_X(1, 1) = X(1, 1);
    new_X(1, 2) = X(1, 2);
    
    %Include sinusoidal terms (1st order)
    new_X(1, 3) = sin(X(1, 1));
    new_X(1, 4) = sin(X(1, 2));
    new_X(1, 5) = cos(X(1, 1));
    new_X(1, 6) = cos(X(1, 2));
%     new_X(1, 7) = sin(X(1, 1).*X(1, 2));
%     new_X(1, 8) = cos(X(1, 1).*X(1, 2));
    
%Include 2nd harmonic sinusoidal terms
    new_X(1, 7) = sin(2*X(1, 1));
    new_X(1, 8) = sin(2*X(1, 2));
    new_X(1, 9) = cos(2*X(1, 1));
    new_X(1, 10) = cos(2*X(1, 2));
    
        %Include 3rd harmonic sinusoidal terms
    new_X(1, 11) = sin(3*X(1, 1));
    new_X(1, 12) = sin(3*X(1, 2));
    new_X(1, 13) = cos(3*X(1, 1));
    new_X(1, 14) = cos(3*X(1, 2));
    
    %Include 4th harmonic sinusoidal terms
    new_X(1, 15) = sin(4*X(1, 1));
    new_X(1, 16) = sin(4*X(1, 2));
    new_X(1, 17) = cos(4*X(1, 1));
    new_X(1, 18) = cos(4*X(1, 2));

%     %Include 2nd order terms
%     new_X(:, 3) = X(:, 1).*X(:, 1);
%     new_X(:, 4) = X(:, 1).*X(:, 2);
%     new_X(:, 5) = X(:, 2).*X(:, 2);
    
%     %Include 3rd order terms
%     new_X(:, 6) = X(:, 1).*X(:, 1).*X(:, 1);
%     new_X(:, 7) = X(:, 1).*X(:, 1).*X(:, 2);
%     new_X(:, 8) = X(:, 1).*X(:, 2).*X(:, 2);
%     new_X(:, 9) = X(:, 2).*X(:, 2).*X(:, 2);
%     
%     %Incluce 4th order terms
%     new_X(:, 10) = X(:, 1).*X(:, 1).*X(:, 1).*X(:, 1);
%     new_X(:, 11) = X(:, 1).*X(:, 1).*X(:, 1).*X(:, 2);
%     new_X(:, 12) = X(:, 1).*X(:, 1).*X(:, 2).*X(:, 2);
%     new_X(:, 13) = X(:, 1).*X(:, 2).*X(:, 2).*X(:, 2);
%     new_X(:, 14) = X(:, 2).*X(:, 2).*X(:, 2).*X(:, 2);
%     
%     %Incluce 5th order terms
%     new_X(:, 15) = X(:, 1).*X(:, 1).*X(:, 1).*X(:, 1).*X(:, 1);
%     new_X(:, 16) = X(:, 1).*X(:, 1).*X(:, 1).*X(:, 1).*X(:, 2);
%     new_X(:, 17) = X(:, 1).*X(:, 1).*X(:, 1).*X(:, 2).*X(:, 2);
%     new_X(:, 18) = X(:, 1).*X(:, 1).*X(:, 2).*X(:, 2).*X(:, 2);
%     new_X(:, 19) = X(:, 1).*X(:, 2).*X(:, 2).*X(:, 2).*X(:, 2);
%     new_X(:, 20) = X(:, 2).*X(:, 2).*X(:, 2).*X(:, 2).*X(:, 2);
%     
%     %Incluce 6th order terms
%     new_X(:, 21) = X(:, 1).*X(:, 1).*X(:, 1).*X(:, 1).*X(:, 1).*X(:, 1);
%     new_X(:, 22) = X(:, 1).*X(:, 1).*X(:, 1).*X(:, 1).*X(:, 1).*X(:, 2);
%     new_X(:, 23) = X(:, 1).*X(:, 1).*X(:, 1).*X(:, 1).*X(:, 2).*X(:, 2);
%     new_X(:, 24) = X(:, 1).*X(:, 1).*X(:, 1).*X(:, 2).*X(:, 2).*X(:, 2);
%     new_X(:, 25) = X(:, 1).*X(:, 1).*X(:, 2).*X(:, 2).*X(:, 2).*X(:, 2);
%     new_X(:, 26) = X(:, 1).*X(:, 2).*X(:, 2).*X(:, 2).*X(:, 2).*X(:, 2);
%     new_X(:, 27) = X(:, 2).*X(:, 2).*X(:, 2).*X(:, 2).*X(:, 2).*X(:, 2);
end

== matlab function MATLAB Simulink Model/Space Vector PWM based VSI /Switching Times and Sector/Angle Calculation1/MATLAB Function ==
  data: wold input; wnew output; wTs input
function wnew = fcn(wold, wTs)
    wnew = rem(wold + wTs, 2*pi);
end

== matlab function MATLAB Simulink Model/Space Vector PWM based VSI /Switching Times and Sector/MATLAB Function2 ==
  data: Vref input; V_alpha output; angle input; V_beta output
function [V_alpha, V_beta] = fcn(Vref, angle)
    V_alpha = Vref*cos(angle);
    V_beta = Vref*sin(angle);
end

== matlab function MATLAB Simulink Model/Space Vector PWM based VSI /Switching Times and Sector/MATLAB Function3 ==
  data: u input; u output
function u = fcn(u)
    u(u<0) = 0;
end

== matlab function MATLAB Simulink Model/Space Vector PWM based VSI /3 Phase VSI/MATLAB Function ==
  data: iter input; iter output; arr input size=[1 3]; Va input; Vb input; Vc input; Ts input; Tsys input; arr output
function [iter, arr] = fcn(iter, arr, Va, Vb, Vc, Ts, Tsys)
    if iter == Ts/Tsys
        iter=0;
        arr = zeros(1,3);
    end
    arr(1, 1) = arr(1, 1) + (Va*Tsys/Ts);
    arr(1, 2) = arr(1, 2) + (Vb*Tsys/Ts);
    arr(1, 3) = arr(1, 3) + (Vc*Tsys/Ts);
    iter = iter+1;
end

== matlab function MATLAB Simulink Model/Space Vector PWM based VSI 1/3 Phase VSI/MATLAB Function ==
  data: iter input; iter output; arr input size=[1 3]; Va input; Vb input; Vc input; Ts input; Tsys input; arr output
function [iter, arr] = fcn(iter, arr, Va, Vb, Vc, Ts, Tsys)
    if iter == Ts/Tsys
        iter=0;
        arr = zeros(1,3);
    end
    arr(1, 1) = arr(1, 1) + (Va*Tsys/Ts);
    arr(1, 2) = arr(1, 2) + (Vb*Tsys/Ts);
    arr(1, 3) = arr(1, 3) + (Vc*Tsys/Ts);
    iter = iter+1;
end

== matlab function MATLAB Simulink Model/Space Vector PWM based VSI /Switching Times and Sector/MATLAB Function4 ==
  data: u input; y output
function y = fcn(u)
    [~, y] = max(u);
end

== matlab function MATLAB Simulink Model/Space Vector PWM based VSI 1/Gate Pulse Generator/Gate Pulse Values ==
  data: count output; count input; G1 output size=1; S1 input; S3 input; S5 input; G3 output size=1; G5 output size=1; Ts input; Tsys input
function [count, G1, G3, G5] = fcn(count, S1, S3, S5, Ts, Tsys)
    count = double(rem(int32(1+count), int32(Ts/Tsys)));
    G1 = S1(1+count);
    G3 = S3(1+count);
    G5 = S5(1+count);
    
%     G1=S1;
%     G3= S3;
%     G5 = S5;
end

== matlab function MATLAB Simulink Model/Space Vector PWM based VSI 1/Gating Pulse Generator/Gate Pulse Generator for 0121 Sequence/For Even Sector/MATLAB Function ==
  data: S1 input; S1 output; S3 input; S5 input; S3 output; S5 output; addtime output; addidx output
function [S1, S3, S5, addtime,addidx] = fcn(S1, S3, S5)
    S = [S1 S3 S5];
    [~, idx] = mink([S1 S3 S5], 3);
    
    addtime = (S(idx(2)) - S(idx(1)))/2;
    addidx = idx(2);
    S(idx(2)) = S(idx(2)) - addtime;
    
    S1 = S(1);
    S3 = S(2);
    S5 = S(3);
end

== matlab function MATLAB Simulink Model/Space Vector PWM based VSI /Switching Times and Sector/m ==
  data: Vref input; m output; Vbus input
function m = fcn(Vref, Vbus)
    m = (2/sqrt(3)) * Vref/Vbus;
end

== matlab function MATLAB Simulink Model/Space Vector PWM based VSI 1/Gating Pulse Generator/Gate Pulse Generator for 0121 Sequence/For Odd Sector/MATLAB Function ==
  data: S1 input; S1 output; S3 input; S5 input; S3 output; S5 output; subtime output; subidx output
function [S1, S3, S5, subtime,subidx] = fcn(S1, S3, S5)
    S = [S1 S3 S5];
    [~, idx] = mink([S1 S3 S5], 3);
    
    S(idx(2)) = (S(idx(2)) + S(idx(3)))/2;
    
    subidx = idx(2);
    subtime = S(idx(3)) - S(idx(2));
    
    S1 = S(1);
    S3 = S(2);
    S5 = S(3);
end

== matlab function MATLAB Simulink Model/Space Vector PWM based VSI 1/Gating Pulse Generator/Gate Pulse Generator for 0127 Sequence 1/For Even Sector/MATLAB Function ==
  data: S1 input; S1 output; S3 input; S5 input; S3 output; S5 output; addtime output; addidx output
function [S1, S3, S5, addtime,addidx] = fcn(S1, S3, S5)
    S = [S1 S3 S5];
    [~, idx] = mink([S1 S3 S5], 3);
    
    addtime = (S(idx(3)) - S(idx(2)))/2;
    addidx = idx(3);
    S(idx(3)) = S(idx(3)) - addtime;
    
    S1 = S(1);
    S3 = S(2);
    S5 = S(3);
end

== matlab function MATLAB Simulink Model/Space Vector PWM based VSI 1/Gating Pulse Generator/Gate Pulse Generator for 0127 Sequence 1/For Odd Sector/MATLAB Function1 ==
  data: S1 input; S1 output; S3 input; S5 input; S3 output; S5 output; subtime output; subidx output
function [S1, S3, S5, subtime,subidx] = fcn(S1, S3, S5)
    S = [S1 S3 S5];
    [~, idx] = mink([S1 S3 S5], 3);
    
    subtime = ( ( S(idx(2)) - S(idx(1)) )/2);
    S(idx(1)) = S(idx(1)) + subtime;
    subidx = idx(1);
    
    S1 = S(1);
    S3 = S(2);
    S5 = S(3);
end

== matlab function MATLAB Simulink Model/Space Vector PWM based VSI 1/Gating Pulse Generator/Gate Pulse Generator for 1012 Sequence/For Even Sector/MATLAB Function1 ==
  data: S1 input; S1 output; S3 input; S5 input; S3 output; S5 output; subtime output; subidx output
function [S1, S3, S5, subtime,subidx] = fcn(S1, S3, S5)
    S = [S1 S3 S5];
    [~, idx] = mink([S1 S3 S5], 3);
    
    subtime = ( ( S(idx(2)) - S(idx(1)) )/2);
    S(idx(1)) = S(idx(1)) + subtime;
    subidx = idx(1);
    
    S1 = S(1);
    S3 = S(2);
    S5 = S(3);
end

== matlab function MATLAB Simulink Model/Space Vector PWM based VSI 1/Gating Pulse Generator/Gate Pulse Generator for 1012 Sequence/For Odd Sector/MATLAB Function ==
  data: S1 input; S1 output; S3 input; S5 input; S3 output; S5 output; addtime output; addidx output
function [S1, S3, S5, addtime,addidx] = fcn(S1, S3, S5)
    S = [S1 S3 S5];
    [~, idx] = mink([S1 S3 S5], 3);
    
    addtime = (S(idx(3)) - S(idx(2)))/2;
    addidx = idx(3);
    S(idx(3)) = S(idx(3)) - addtime;
    
    S1 = S(1);
    S3 = S(2);
    S5 = S(3);
end

== matlab function MATLAB Simulink Model/Space Vector PWM based VSI 1/Gating Pulse Generator/Gate Pulse Generator for 2721 Sequence/For Even Sector/MATLAB Function ==
  data: S1 input; S1 output; S3 input; S5 input; S3 output; S5 output; addtime output; addidx output
function [S1, S3, S5, addtime,addidx] = fcn(S1, S3, S5)
    S = [S1 S3 S5];
    [~, idx] = mink([S1 S3 S5], 3);
    
    addtime = (S(idx(3)) - S(idx(2)))/2;
    addidx = idx(3);
    S(idx(3)) = S(idx(3)) - addtime;
    
    S1 = S(1);
    S3 = S(2);
    S5 = S(3);
end

== matlab function MATLAB Simulink Model/Space Vector PWM based VSI 1/Gating Pulse Generator/Gate Pulse Generator for 2721 Sequence/For Odd Sector/MATLAB Function1 ==
  data: S1 input; S1 output; S3 input; S5 input; S3 output; S5 output; subtime output; subidx output
function [S1, S3, S5, subtime,subidx] = fcn(S1, S3, S5)
    S = [S1 S3 S5];
    [~, idx] = mink([S1 S3 S5], 3);
    
    subtime = ( ( S(idx(2)) - S(idx(1)) )/2);
    S(idx(1)) = S(idx(1)) + subtime;
    subidx = idx(1);
    
    S1 = S(1);
    S3 = S(2);
    S5 = S(3);
end

== matlab function MATLAB Simulink Model/RMS Error Calculation /Subsystem/MATLAB Function ==
  data: phi_d_rms input; prev_it_num input; phi_d input; phi_d_rms output; curr_it_num output; Ts input; Tsys input
function [phi_d_rms, curr_it_num]= fcn(phi_d_rms, prev_it_num, phi_d, Ts, Tsys)
curr_it_num = prev_it_num+1;

if  int16(curr_it_num) == int16(Ts/Tsys)
    phi_d_rms=0;
    curr_it_num = 1;
end

phi_d_rms = phi_d_rms + (abs(phi_d)*abs(phi_d)*Tsys);
end

== matlab function MATLAB Simulink Model/Space Vector PWM based VSI 1/Gating Pulse Generator/Gate Pulse Generator for 7212 Sequence/For Even Sector/MATLAB Function1 ==
  data: S1 input; S1 output; S3 input; S5 input; S3 output; S5 output; subtime output; subidx output
function [S1, S3, S5, subtime,subidx] = fcn(S1, S3, S5)
    S = [S1 S3 S5];
    [~, idx] = mink([S1 S3 S5], 3);
    
    S(idx(2)) = (S(idx(2)) + S(idx(3)))/2;
    
    subidx = idx(2);
    subtime = S(idx(3)) - S(idx(2));
    
    S1 = S(1);
    S3 = S(2);
    S5 = S(3);
end

== matlab function MATLAB Simulink Model/Space Vector PWM based VSI 1/Gating Pulse Generator/Gate Pulse Generator for 7212 Sequence/For Odd Sector/MATLAB Function ==
  data: S1 input; S1 output; S3 input; S5 input; S3 output; S5 output; addtime output; addidx output
function [S1, S3, S5, addtime,addidx] = fcn(S1, S3, S5)
    S = [S1 S3 S5];
    [~, idx] = mink([S1 S3 S5], 3);
    
    addtime = (S(idx(2)) - S(idx(1)))/2;
    addidx = idx(2);
    S(idx(2)) = S(idx(2)) - addtime;
    
    S1 = S(1);
    S3 = S(2);
    S5 = S(3);
end

== matlab function MATLAB Simulink Model/Space Vector PWM based VSI 1/Switching Times and Sector/Angle Calculation1/MATLAB Function ==
  data: wold input; wnew output; wTs input
function wnew = fcn(wold, wTs)
    wnew = rem(wold + wTs, 2*pi);
end

== matlab function MATLAB Simulink Model/Space Vector PWM based VSI 1/Switching Times and Sector/Switch Times and Sequence Calculation ==
  data: S1 output; S3 output; S5 output; Vref input; angle input; Ts input; Vbus input; sector output; swseq output
function [S1, S3, S5, sector, swseq] = fcn(Vref, angle, Ts, Vbus)
    numzones = 5;
    %     Method 2 
    m = (2/sqrt(3))*(Vref/Vbus);
    theta = rem(angle, (pi/3));
    flag = 0;
    if numzones == 1
        flag = 1;
    end
    
    %Switching times calculation of different vectors
    if m <= 1                % Linear modulation (Overmodulation mode 0)
        n2 = Vref*cos( theta );
        n1 = Vref*cos( (pi/3) - theta );

        T1 = (2*Ts/(3*Vbus)) * ((-n1) + (2*n2));
        T2 = (2*Ts/(3*Vbus)) * ((2*n1) - n2);
        T0 = Ts-(T1+T2);
        flag = 1;
        
    elseif m<=1.05      % Overmodulation mode I
        alpha_t = (pi/6) - acos(1/m);
        alpha_t = alpha_t/2;
        if theta > alpha_t && theta < (pi/3) - alpha_t
            T1 = (sin( (pi/3) - theta ) / ( sin( (pi/3) - theta ) + sin( theta ) ) ) * Ts;
            T2 = Ts-T1;
            T0=0;
        else
            n2 = Vref*cos( theta );
            n1 = Vref*cos( (pi/3) - theta );
            T1 = (2*Ts/(3*Vbus)) * ((-n1) + (2*n2));
            T2 = (2*Ts/(3*Vbus)) * ((2*n1) - n2);
            T0 = Ts-(T1+T2);
            flag = 1;
        end
        
    elseif m <= 1.10    % Overmodulation mode II
        alpha_h = (pi/6) - acos(1/m);
        if theta <= alpha_h
            T1 = Ts;
            T2=0;
            T0=0;
            
        elseif theta > alpha_h && theta < (pi/3) - alpha_h
            T1 = (sin( (pi/3) - theta ) / ( sin( (pi/3) - theta ) + sin( theta ) ) ) * Ts;
            T2 = Ts-T1;
            T0=0;
            
        else
            T1 = 0;
            T2 = Ts;
            T0 = 0;
        end
        
    else        % Six Step Mode
        if theta <= (pi/6)
            T1 = Ts;
            T2 = 0;
            T0 = 0;
        else
            T1 = 0;
            T2 = Ts;
            T0 = 0;
        end
        
    end
    
    if flag == 1
        % Switching Sequence Determination
        Q1 = (cos(theta) - (Vref/Vbus)) * T1;
        Q2 = (cos( (pi/3) - theta) - (Vref/Vbus)) * T2;
        Q0 = - (Vref/Vbus)*T0;
        D = sin(theta) * T1;

        %Error Functions (Squared) for Different Switching Sequences
        F_0127 = ( (1/3) * ( (0.5*Q0).^2 ) * T0 / (2*Ts) ) + ( (1/3) * ( ( (0.5*Q0).^2 ) + ( 0.5*Q0* ( (0.5*Q0) + Q1 ) ) + ( ( 1* ( (0.5*Q0) + Q1 ) ).^2) ) * (T1/Ts) ) + ( (1/3) * ( ( ( (0.5*Q0) + Q1).^2) - ( ( (0.5*Q0) + Q1) * (0.5*Q0) ) + ( (0.5*Q0).^2 ) ) * (T2/Ts) ) + ( (1/3) * ( (0.5*Q0).^2 ) * ( T0 / (2*Ts) ) ) + ( (1/3) * (D.^2) * ( (T1+T2) / Ts ) );

        F_012 = ( (4/27) * (Q0.^2) * (T0/Ts) ) + ( (4/27) * ( (Q0.^2) + ( Q0*(Q0+Q1) ) + ( (Q0+Q1).^2 ) ) * (T1/Ts) ) + ( (4/27) * ( (Q0+Q1).^2 ) * (T2/Ts) ) + ( (4/27) * (D.^2) * ( (T1+T2) / Ts) );

        F_721 = ( (4/27) * (Q0.^2) * (T0/Ts) ) + ( (4/27) * ( (Q0.^2) + ( Q0*(Q0+Q2) ) + ( (Q0+Q2).^2 ) ) * (T2/Ts) ) + ( (4/27) * ( (Q0+Q2).^2 ) * (T1/Ts) ) + ( (4/27) * (D.^2) * ( (T1+T2) / Ts) );

        F_0121 = ( (1/3) * (Q0.^2) * (T0/Ts) ) + ( (1/3) * ( (Q0.^2) + ( Q0*( Q0 + (0.5*Q1) ) ) + ( ( Q0 + (0.5*Q1) ).^2 ) ) * ( T1 / (2*Ts) ) ) + ( (1/3) * ( ( ( Q0 + (0.5*Q1) ).^2 ) - ( ( Q0 + (0.5*Q1) ) * (0.5*Q1) ) + ( (0.5*Q1).^2 ) ) * (T2/Ts) ) + ( (1/3) * ( (0.5*Q1).^2 ) * (T1 / (2*Ts) ) ) + ( (1/3) * ( (0.5*D).^2 ) * ( (T1+T2) / Ts ) );

        F_7212 = ( (1/3) * (Q0.^2) * (T0/Ts) ) + ( (1/3) * ( (Q0.^2) + ( Q0*( Q0 + (0.5*Q2) ) ) + ( ( Q0 + (0.5*Q2) ).^2 ) ) * ( T2 / (2*Ts) ) ) + ( (1/3) * ( ( ( Q0 + (0.5*Q2) ).^2 ) - ( ( Q0 + (0.5*Q2) ) * (0.5*Q2) ) + ( (0.5*Q2).^2 ) ) * (T1/Ts) ) + ( (1/3) * ( (0.5*Q2).^2 ) * (T2 / (2*Ts) ) ) + ( (1/3) * ( (0.5*D).^2 ) * ( (T1+T2) / Ts ) );

        F_1012 = ( (1/3) * ( ( 0.5*Q1).^2 ) * (T1 / (2*Ts) ) ) + ( (1/3) * ( ( (0.5*Q1).^2 ) + ( 0.5*Q1*( (0.5*Q1) + Q0 ) ) + ( ( (0.5*Q1) + Q0 ).^2 ) ) * (T0/Ts) ) + ( (1/3) * ( ( ( (0.5*Q1) + Q0 ).^2 ) - ( ( (0.5*Q1) + Q0 )*Q2 ) + (Q2.^2) ) * ( T1 / (2*Ts) ) ) + ( (1/3) * (Q2.^2) * (T2/Ts) ) + ( (1/3) * ( (0.5*D).^2 ) * ( T1 / (2*Ts) ) ) + ( ( (0.5*D).^2 ) * (T0/Ts) ) + ( (1/3) * ( ( (0.5*D).^2 ) + ( (0.5*D) * D ) + (D.^2) ) * ( T1 / (2*Ts) ) ) + ( (1/3) * (D.^2) * (T2/Ts) );

        F_2721 = ( (1/3) * ( ( 0.5*Q2).^2 ) * (T2 / (2*Ts) ) ) + ( (1/3) * ( ( (0.5*Q2).^2 ) + ( 0.5*Q2*( (0.5*Q2) + Q0 ) ) + ( ( (0.5*Q2) + Q0 ).^2 ) ) * (T0/Ts) ) + ( (1/3) * ( ( ( (0.5*Q2) + Q0 ).^2 ) - ( ( (0.5*Q2) + Q0 )*Q1 ) + (Q1.^2) ) * ( T2 / (2*Ts) ) ) + ( (1/3) * (Q1.^2) * (T1/Ts) ) + ( (1/3) * ( (0.5*D).^2 ) * ( T2 / (2*Ts) ) ) + ( ( (0.5*D).^2 ) * (T0/Ts) ) + ( (1/3) * ( ( (0.5*D).^2 ) + ( (0.5*D) * D ) + (D.^2) ) * ( T2 / (2*Ts) ) ) + ( (1/3) * (D.^2) * (T1/Ts) );
        
        if numzones == 1
            F = [F_0127];
            
        elseif numzones == 3
            %For Three Zone Hybrid PWM
            F = [F_0127, F_0121, F_7212];
            
        elseif numzones == 5
            %For Five Zone Hybrid PWM
            F = [F_0127, F_0121, F_7212, F_1012, F_2721];
        
        elseif numzones == 7
            %For Seven Zone Hybrid PWM
            F = [F_0127, F_0121, F_7212, F_1012, F_2721, F_012, F_721];
            
        else
            F = F_0127;
        end
        
        [~, idx] = min(F);

        if idx == 1
            switchseq = "0127";
        elseif idx == 2
            switchseq = "0121";
        elseif idx == 3
            switchseq = "7212";
        elseif idx == 4
            switchseq = "1012";
        elseif idx == 5
            switchseq = "2721";
        elseif idx == 6
            switchseq = "012";
        elseif idx == 7
            switchseq = "721";
        else
            switchseq = "0127";
        end
        
    else
        if theta < (pi/6)
            switchseq = "0121";
        else
            switchseq = "7212";
        end
    end
%     switchseq = "0127";
    % Switching Times calculation of switches
    Vsamp = Vref*exp(1i*angle);
    
    V1 = Vbus*exp(1i*0);
    V2 = Vbus*exp(1i*(pi/3));
    V3 = Vbus*exp(1i*(2*pi/3));
    V4 = Vbus*exp(1i*(3*pi/3));
    V5 = Vbus*exp(1i*(4*pi/3));
    V6 = Vbus*exp(1i*(5*pi/3));

    V = [V1; V2; V3; V4; V5; V6];
    V = V - Vsamp;
    [~, minVidx] = mink(V, 2);

%         minVidx = minVidx(:, 1);

    if max(minVidx) == 6 && min(minVidx) == 1
        minVidx = 6;
    else
        minVidx = min(minVidx);
    end
    
    Gmax = 0;
    Gmed = 0;
    Glow = 0;
    if switchseq == "0127"
        Gmax = T1+T2+(T0/2);
        if rem(minVidx, 2) == 1
            Gmed = T2 + (T0/2);
        else
            Gmed = T1 + (T0/2);
        end
        Glow = (T0/2);
        
    elseif switchseq == "0121" || switchseq == "1012" || switchseq == "012"
        if rem(minVidx, 2) == 1 
            Gmax = T1+T2;
            Gmed = T2;
            Glow = 0;
        else 
            Gmax = T1+T2+T0;
            Gmed = T1+T0;
            Glow = T0;
        end
        
    elseif switchseq == "7212" || switchseq == "2721" || switchseq == "721"
        if rem(minVidx, 2) == 1
            Gmax = T1+T2+T0;
            Gmed = T2+T0;
            Glow = T0;
        else
            Gmax = T1+T2;
            Gmed = T1;
            Glow = 0;
        end
        
    end
    
%     timings = zeros(6, 3, int32(Ts/Tsys));
    timings = zeros(6, 3);
    timings(1, :) = [Gmax        ;     Gmed        ;     Glow         ];
    timings(2, :) = [Gmed        ;     Gmax        ;     Glow         ];
    timings(3, :) = [Glow         ;     Gmax        ;     Gmed        ];
    timings(4, :) = [Glow         ;     Gmed        ;     Gmax        ];
    timings(5, :) = [Gmed        ;     Glow         ;     Gmax        ];
    timings(6, :) = [Gmax        ;     Glow         ;     Gmed        ];
    
    answ = squeeze(real(timings(minVidx, :)));
%     size(answ)
    
    S1 = answ(1);
%     S1 = S1(:);
    S3 = answ(2);
%     S3 = S3(:);
    S5 = answ(3);
%     S5 = S5(:);
    sector = minVidx;
    
    if switchseq == "0127"
        swseq = 1;
    elseif switchseq == "0121"
        swseq = 2;
    elseif switchseq == "7212"
        swseq = 3;
    elseif switchseq == "1012"
        swseq = 4;
    elseif switchseq == "2721"
        swseq = 5;
    elseif switchseq == "012"
        swseq = 6;
    elseif switchseq == "721"
        swseq = 7;
    else
        swseq = 1;
    end
%     if swseq == 5
%         swseq = 3;
%     end
end
